simulink model "F16_dynamic_model_2019a"  (R2024b)
settings: Solver=ode3  StartTime=0.0  StopTime=1  FixedStep=1/1000  RelTol=1e-3
values from neighbouring files (symbols this model uses):
  f16data =     [f16aerodata.mat]
  f16engine =     [f16engine.mat]
undefined symbols (not defined in the file or in its folder): e0_0, e1_0, e2_0, e3_0, Earth, ft, m, s, WGS84
libraries: simulink_extras x11, simulink x7, aerosimlib x5, vrlib x3, sharedtransform x3, aerolibfltsims x3, slpidlib x3, aerolibconvert2 x2, aerolibutil x1, sharedutil x1, shared6dof x1, aerolibtransform2 x1
(part 1 of 3)
settings Model: SimulationMode=accelerator  PauseTimes=2  Creator=PC_2565  LastModifiedBy=MSI
settings SolverCC: AlgebraicLoopSolver=TrustRegion
settings DebuggingCC: UnconnectedInputMsg=warning  UnconnectedOutputMsg=warning  UnconnectedLineMsg=warning
settings ModelReferenceCC: EnableRefExpFcnMdlSchedulingChecks=on
settings SFSimCC: CustomCodeUndefinedFunction=UseInterfaceOnly
settings RTWCC: GPUComputeCapability=3.5

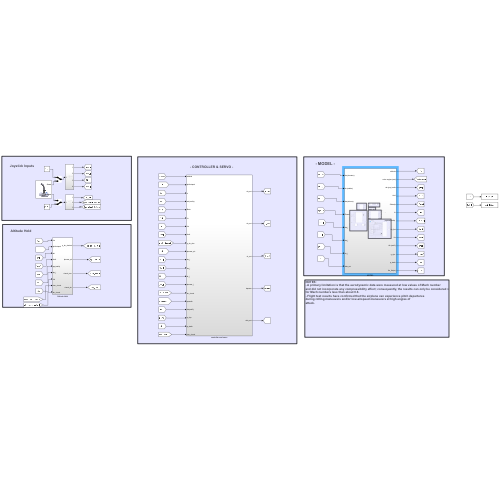
[thumbnail: Simulink's stored preview of the top-level diagram]
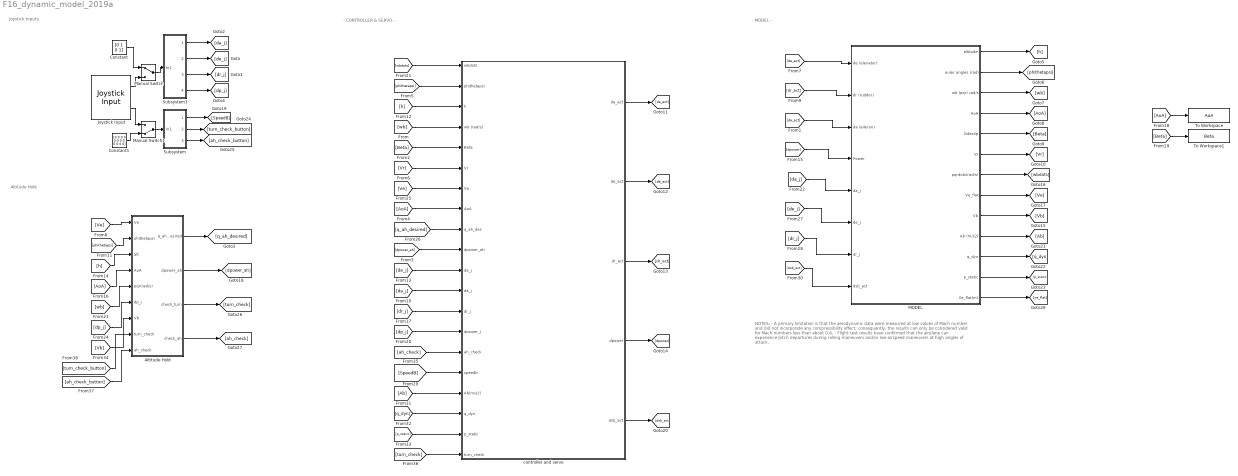
== system F16_dynamic_model_2019a ==
  note: NOTES:
      | - A primary limitation is that the aerodynamic data were measured at low values of Mach number
      | and did not incorporate any compressibility effect; consequently, the results can only be considered valid
      | for Mach numbers less than about 0.6.
      | - Flight test results have confirmed that the airplane can experience pitch departures
      | during rolling maneuvers and/or low-airspeed maneuvers at high angles of
      | attack.
  note: - CONTROLLER & SERVO -
  note: Altitude Hold
  note: Joystick Inputs
  note: - MODEL -
  Altitude Hold : Subsystem
  Constant : Constant  Value=[0 1 0 1]
  Constant1 : Constant  Value=[0 0 0 0 0 0 0 0 0 0 0 0]
  Joystick Input : vrlib/Joystick Input  joyid=1  adjustports=on  forcefeed=off
  MODEL : Subsystem
  Manual Switch : ManualSwitch
  Manual Switch1 : ManualSwitch  CurrentSetting=0
  Subsystem : Subsystem
  Subsystem3 : Subsystem
  To Workspace : ToWorkspace  VariableName=AoA  SampleTime=-1
  To Workspace1 : ToWorkspace  VariableName=Beta  SampleTime=-1
      settings: Save2DSignal=2-D array (concatenate along first dimension)
  "controller and servo " : Subsystem
  wires:
  Subsystem3/3(Out3) -> [dr_j]
  Subsystem3/4(Out4) -> [dp_j]
  MODEL/1(altitude) -> [h]
  MODEL/2(euler angles (rad)) -> [phithetapsi]
  MODEL/4(AoA) -> [AoA]
  MODEL/3(wb (pqr) rad/s) -> [wb]
  MODEL/5(Sideslip) -> [Beta]
  MODEL/6(Vr) -> [Vr]
  [phithetapsi] -> "controller and servo "/2(phithetapsi)
  "controller and servo "/1(da_act) -> [da_act]
  "controller and servo "/3(dr_act) -> [dr_act]
  [Vr] -> "controller and servo "/6(Vr)
  "controller and servo "/4(dpower) -> [dpower]
  [AoA] -> "controller and servo "/8(AoA)
  [h] -> "controller and servo "/3(h)
  [wb] -> "controller and servo "/4(wb (rad/s))
  MODEL/9(Vb) -> [Vb]
  [Ve] -> "controller and servo "/7(Ve)
  [Beta] -> "controller and servo "/5("Beta ")
  [AoA] -> To Workspace/1
  [Beta] -> To Workspace1/1
  [da_j] -> "controller and servo "/12(da_j)
  [de_j] -> "controller and servo "/11(de_j)
  [dr_j] -> "controller and servo "/13(dr_j)
  [dp_j] -> "controller and servo "/14(dpower_j)
  "controller and servo "/2(de_act) -> [de_act]
  [phithetapsi] -> Altitude Hold/2(phithetapsi)
  [h] -> Altitude Hold/3(alt)
  [AoA] -> Altitude Hold/4(AoA)
  [de_act] -> MODEL/1(de (elevator))
  [da_act] -> MODEL/3(da (aileron))
  [dr_act] -> MODEL/2(dr (rudder))
  [dpower] -> MODEL/4(Power)
  MODEL/7("pqrdots(rad/s) ") -> [wbdots]
  [wbdots] -> "controller and servo "/1(wbdots)
  [Ve] -> Altitude Hold/1(Ve)
  [wb] -> Altitude Hold/5(pqr(rad/s))
  [dp_j] -> Altitude Hold/6(dp_j)
  [ah_check] -> "controller and servo "/15("ah_check ")
  MODEL/8(Ve_flat) -> [Ve]
  Altitude Hold/1(q_ah_desired) -> [q_ah_desired]
  Altitude Hold/2(dpower_ah) -> [dpower_ah]
  [dpower_ah] -> "controller and servo "/10(dpower_ah)
  [q_ah_desired] -> "controller and servo "/9(q_ah_des)
  Joystick Input/1 -> Manual Switch/2
  Subsystem3/1(Out1) -> [da_j]
  Subsystem3/2(Out2) -> [de_j]
  [da_j] -> MODEL/5(da_j)
  [de_j] -> MODEL/6(de_j)
  [dr_j] -> MODEL/7(dr_j)
  [SpeedB] -> "controller and servo "/16(speedb)
  "controller and servo "/5(dsb_act) -> [dsb_act]
  [dsb_act] -> MODEL/8(dsb_act)
  MODEL/10(Ab (m/s2)) -> [Ab]
  [Ab] -> "controller and servo "/17(Ab(m/s2))
  MODEL/11("q_dyn ") -> [q_dyn]
  [q_dyn] -> "controller and servo "/18(q_dyn)
  MODEL/12(p_static) -> [p_static]
  [p_static] -> "controller and servo "/19(p_static)
  [Vb] -> Altitude Hold/7(Vb)
  Joystick Input/2 -> Manual Switch1/1
  Subsystem/1(Out1) -> [SpeedB]
  Subsystem/2(Out2) -> [turn_check_button]
  Subsystem/3(Out3) -> [ah_check_button]
  [turn_check] -> "controller and servo "/20("turn_check ")
  [turn_check_button] -> Altitude Hold/8("turn_check ")
  Altitude Hold/3("check_turn ") -> [turn_check]
  [ah_check_button] -> Altitude Hold/9(ah_check)
  Altitude Hold/4("check_ah ") -> [ah_check]
  Constant/1 -> Manual Switch/1
  Constant1/1 -> Manual Switch1/2
  MODEL/13(Xe_flat(m)) -> [xe_flat]
  Manual Switch1/1 -> Subsystem/1(In1)
  Manual Switch/1 -> Subsystem3/1(In1)

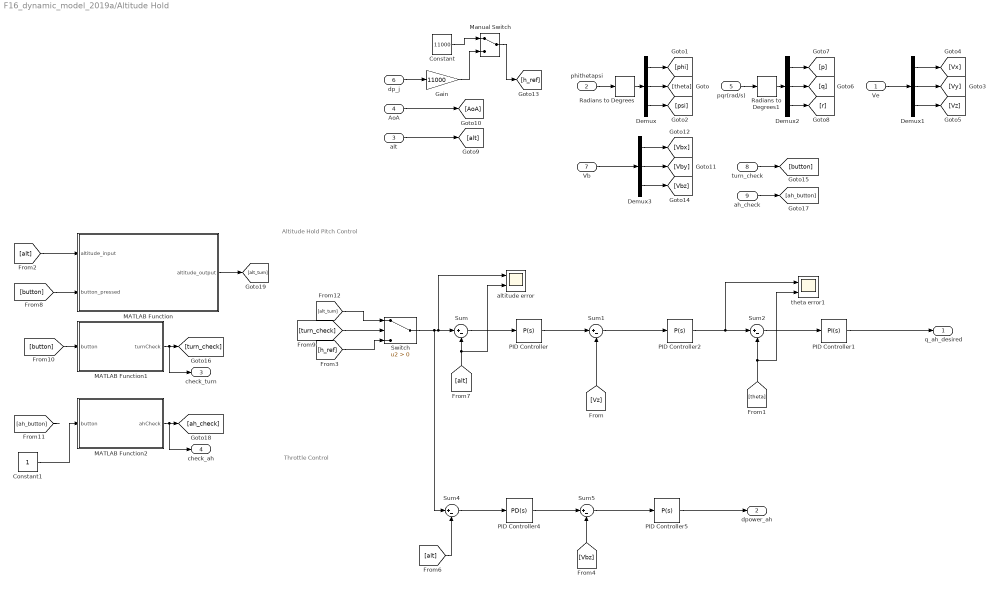
== system F16_dynamic_model_2019a/Altitude Hold ==
  note: Throttle Control
  note: Altitude Hold Pitch Control
  Ve : Inport
  phithetapsi : Inport  Port=2
  alt : Inport  Port=3
  AoA : Inport  Port=4
  pqr(rad/s) : Inport  Port=5
  dp_j : Inport  Port=6
  Vb : Inport  Port=7
  "turn_check " : Inport  Port=8
  ah_check : Inport  Port=9
  Constant : Constant  Value=11000
  Constant1 : Constant
  Demux{,1..3} (4 alike) : Demux  Outputs=3
  Gain : Gain  Gain=11000
  MATLAB Function : MATLAB Function  TreatAsAtomicUnit=on
  MATLAB Function1 : MATLAB Function  TreatAsAtomicUnit=on
  MATLAB Function2 : MATLAB Function  TreatAsAtomicUnit=on
  Manual Switch : ManualSwitch
  PID Controller : simulink/Continuous/PID Controller  Controller=P  Form=Parallel  TimeDomain=Continuous-time  SampleTime=-1  IntegratorMethod=Forward Euler  FilterMethod=Forward Euler  ControllerParametersSource=internal  P=2  I=0.00000001  D=10  UseFilter=on  N=100  TunerSelectOption=Transfer Function Based (PID Tuner App)  InitialConditionSource=internal  InitialConditionForIntegrator=0  InitialConditionForFilter=0  DifferentiatorICPrevScaledInput=0  ExternalReset=none  TrackingMode=off  Kt=1  LimitOutput=on  UpperSaturationLimit=254  LowerSaturationLimit=-254  LinearizeAsGain=on  AntiWindupMode=none  Kb=1  POutMin=[]  POutMax=[]  IOutMin=[]  IOutMax=[]  DOutMin=[]  DOutMax=[]  NOutMin=[]  NOutMax=[]  SumOutMin=[]  SumOutMax=[]  SaturationOutMin=[]  SaturationOutMax=[]  PParamMin=[]  PParamMax=[]  IParamMin=[]  IParamMax=[]  DParamMin=[]  DParamMax=[]  NParamMin=[]  NParamMax=[]  KbParamMin=[]  KbParamMax=[]  KtParamMin=[]  KtParamMax=[]  KbOutMin=[]  KbOutMax=[]  KtOutMin=[]  KtOutMax=[]  IntegratorOutMin=[]  IntegratorOutMax=[]  FilterOutMin=[]  FilterOutMax=[]  SumI1OutMin=[]  SumI1OutMax=[]  SumI2OutMin=[]  SumI2OutMax=[]  SumI3OutMin=[]  SumI3OutMax=[]  SumI4OutMin=[]  SumI4OutMax=[]  SumDOutMin=[]  SumDOutMax=[]  DifferentiatorOutMin=[]  DifferentiatorOutMax=[]  FilterDiffOutCoefMin=[]  FilterDiffOutCoefMax=[]  ReciprocalOutMin=[]  ReciprocalOutMax=[]  SumDenOutMin=[]  SumDenOutMax=[]  SumNumOutMin=[]  SumNumOutMax=[]  DivideOutMin=[]  DivideOutMax=[]  IntegratorContinuousStateAttributes=''  IntegratorStateMustResolveToSignalObject=off  IntegratorRTWStateStorageClass=Auto  FilterContinuousStateAttributes=''  FilterStateMustResolveToSignalObject=off  FilterRTWStateStorageClass=Auto  ParallelPVariant=InternalParameters  IdealPVariant=Disabled  IVariant=Disabled  DVariant=Disabled  IntegratorVariant=Disabled  SatVariant=Enabled  AWVariant=Disabled  PCopyVariant=Disabled  TRVariant=Disabled  FdbkBlocksVariant=Forward  IdealPFdbkVariant=Disabled  SatFdbkVariant=Disabled  DerivativeFilterVariant=Disabled  NVariant=Disabled  NCopyVariant=Disabled_SignalSpec  FilterICVariant=Disabled  IntegratorICVariant=Disabled  ExternalResetVariant=Disabled  TRSumVariant=Passthrough  SumFdbkVariant=Disabled  SumVariant=Passthrough_P
  PID Controller1 : simulink/Continuous/PID Controller  Controller=PI  Form=Parallel  TimeDomain=Continuous-time  SampleTime=-1  IntegratorMethod=Forward Euler  FilterMethod=Forward Euler  ControllerParametersSource=internal  P=0.1  I=0.01  D=10  UseFilter=on  N=100  TunerSelectOption=Transfer Function Based (PID Tuner App)  InitialConditionSource=internal  InitialConditionForIntegrator=0  InitialConditionForFilter=0  DifferentiatorICPrevScaledInput=0  ExternalReset=none  TrackingMode=off  Kt=1  LimitOutput=on  UpperSaturationLimit=inf  LowerSaturationLimit=-inf  LinearizeAsGain=on  AntiWindupMode=clamping  Kb=1  POutMin=[]  POutMax=[]  IOutMin=[]  IOutMax=[]  DOutMin=[]  DOutMax=[]  NOutMin=[]  NOutMax=[]  SumOutMin=[]  SumOutMax=[]  SaturationOutMin=[]  SaturationOutMax=[]  PParamMin=[]  PParamMax=[]  IParamMin=[]  IParamMax=[]  DParamMin=[]  DParamMax=[]  NParamMin=[]  NParamMax=[]  KbParamMin=[]  KbParamMax=[]  KtParamMin=[]  KtParamMax=[]  KbOutMin=[]  KbOutMax=[]  KtOutMin=[]  KtOutMax=[]  IntegratorOutMin=[]  IntegratorOutMax=[]  FilterOutMin=[]  FilterOutMax=[]  SumI1OutMin=[]  SumI1OutMax=[]  SumI2OutMin=[]  SumI2OutMax=[]  SumI3OutMin=[]  SumI3OutMax=[]  SumI4OutMin=[]  SumI4OutMax=[]  SumDOutMin=[]  SumDOutMax=[]  DifferentiatorOutMin=[]  DifferentiatorOutMax=[]  FilterDiffOutCoefMin=[]  FilterDiffOutCoefMax=[]  ReciprocalOutMin=[]  ReciprocalOutMax=[]  SumDenOutMin=[]  SumDenOutMax=[]  SumNumOutMin=[]  SumNumOutMax=[]  DivideOutMin=[]  DivideOutMax=[]  IntegratorContinuousStateAttributes=''  IntegratorStateMustResolveToSignalObject=off  IntegratorRTWStateStorageClass=Auto  FilterContinuousStateAttributes=''  FilterStateMustResolveToSignalObject=off  FilterRTWStateStorageClass=Auto  ParallelPVariant=InternalParameters  IdealPVariant=Disabled  IVariant=InternalParameters  DVariant=Disabled  IntegratorVariant=Continuous  SatVariant=Enabled  AWVariant=ContClampingParallel  PCopyVariant=Disabled  TRVariant=Disabled  FdbkBlocksVariant=Forward  IdealPFdbkVariant=Disabled  SatFdbkVariant=Disabled  DerivativeFilterVariant=Disabled  NVariant=Disabled  NCopyVariant=Disabled_SignalSpec  FilterICVariant=Disabled  IntegratorICVariant=InternalICs  ExternalResetVariant=Disabled  TRSumVariant=Passthrough  SumFdbkVariant=Disabled  SumVariant=Sum_PI
  PID Controller2 : simulink/Continuous/PID Controller  Controller=P  Form=Parallel  TimeDomain=Continuous-time  SampleTime=-1  IntegratorMethod=Forward Euler  FilterMethod=Forward Euler  ControllerParametersSource=internal  P=2  I=0.001  D=0.1  UseFilter=on  N=100  TunerSelectOption=Transfer Function Based (PID Tuner App)  InitialConditionSource=internal  InitialConditionForIntegrator=0  InitialConditionForFilter=0  DifferentiatorICPrevScaledInput=0  ExternalReset=none  TrackingMode=off  Kt=1  LimitOutput=on  UpperSaturationLimit=45  LowerSaturationLimit=-45  LinearizeAsGain=on  AntiWindupMode=none  Kb=1  POutMin=[]  POutMax=[]  IOutMin=[]  IOutMax=[]  DOutMin=[]  DOutMax=[]  NOutMin=[]  NOutMax=[]  SumOutMin=[]  SumOutMax=[]  SaturationOutMin=[]  SaturationOutMax=[]  PParamMin=[]  PParamMax=[]  IParamMin=[]  IParamMax=[]  DParamMin=[]  DParamMax=[]  NParamMin=[]  NParamMax=[]  KbParamMin=[]  KbParamMax=[]  KtParamMin=[]  KtParamMax=[]  KbOutMin=[]  KbOutMax=[]  KtOutMin=[]  KtOutMax=[]  IntegratorOutMin=[]  IntegratorOutMax=[]  FilterOutMin=[]  FilterOutMax=[]  SumI1OutMin=[]  SumI1OutMax=[]  SumI2OutMin=[]  SumI2OutMax=[]  SumI3OutMin=[]  SumI3OutMax=[]  SumI4OutMin=[]  SumI4OutMax=[]  SumDOutMin=[]  SumDOutMax=[]  DifferentiatorOutMin=[]  DifferentiatorOutMax=[]  FilterDiffOutCoefMin=[]  FilterDiffOutCoefMax=[]  ReciprocalOutMin=[]  ReciprocalOutMax=[]  SumDenOutMin=[]  SumDenOutMax=[]  SumNumOutMin=[]  SumNumOutMax=[]  DivideOutMin=[]  DivideOutMax=[]  IntegratorContinuousStateAttributes=''  IntegratorStateMustResolveToSignalObject=off  IntegratorRTWStateStorageClass=Auto  FilterContinuousStateAttributes=''  FilterStateMustResolveToSignalObject=off  FilterRTWStateStorageClass=Auto  ParallelPVariant=InternalParameters  IdealPVariant=Disabled  IVariant=Disabled  DVariant=Disabled  IntegratorVariant=Disabled  SatVariant=Enabled  AWVariant=Disabled  PCopyVariant=Disabled  TRVariant=Disabled  FdbkBlocksVariant=Forward  IdealPFdbkVariant=Disabled  SatFdbkVariant=Disabled  DerivativeFilterVariant=Disabled  NVariant=Disabled  NCopyVariant=Disabled_SignalSpec  FilterICVariant=Disabled  IntegratorICVariant=Disabled  ExternalResetVariant=Disabled  TRSumVariant=Passthrough  SumFdbkVariant=Disabled  SumVariant=Passthrough_P
  PID Controller4 : simulink/Continuous/PID Controller  Controller=PD  Form=Parallel  TimeDomain=Continuous-time  SampleTime=-1  IntegratorMethod=Forward Euler  FilterMethod=Forward Euler  ControllerParametersSource=internal  P=5  I=0.00000001  D=10  UseFilter=on  N=100  TunerSelectOption=Transfer Function Based (PID Tuner App)  InitialConditionSource=internal  InitialConditionForIntegrator=0  InitialConditionForFilter=0  DifferentiatorICPrevScaledInput=0  ExternalReset=none  TrackingMode=off  Kt=1  LimitOutput=on  UpperSaturationLimit=254  LowerSaturationLimit=-254  LinearizeAsGain=on  AntiWindupMode=none  Kb=1  POutMin=[]  POutMax=[]  IOutMin=[]  IOutMax=[]  DOutMin=[]  DOutMax=[]  NOutMin=[]  NOutMax=[]  SumOutMin=[]  SumOutMax=[]  SaturationOutMin=[]  SaturationOutMax=[]  PParamMin=[]  PParamMax=[]  IParamMin=[]  IParamMax=[]  DParamMin=[]  DParamMax=[]  NParamMin=[]  NParamMax=[]  KbParamMin=[]  KbParamMax=[]  KtParamMin=[]  KtParamMax=[]  KbOutMin=[]  KbOutMax=[]  KtOutMin=[]  KtOutMax=[]  IntegratorOutMin=[]  IntegratorOutMax=[]  FilterOutMin=[]  FilterOutMax=[]  SumI1OutMin=[]  SumI1OutMax=[]  SumI2OutMin=[]  SumI2OutMax=[]  SumI3OutMin=[]  SumI3OutMax=[]  SumI4OutMin=[]  SumI4OutMax=[]  SumDOutMin=[]  SumDOutMax=[]  DifferentiatorOutMin=[]  DifferentiatorOutMax=[]  FilterDiffOutCoefMin=[]  FilterDiffOutCoefMax=[]  ReciprocalOutMin=[]  ReciprocalOutMax=[]  SumDenOutMin=[]  SumDenOutMax=[]  SumNumOutMin=[]  SumNumOutMax=[]  DivideOutMin=[]  DivideOutMax=[]  IntegratorContinuousStateAttributes=''  IntegratorStateMustResolveToSignalObject=off  IntegratorRTWStateStorageClass=Auto  FilterContinuousStateAttributes=''  FilterStateMustResolveToSignalObject=off  FilterRTWStateStorageClass=Auto  ParallelPVariant=InternalParameters  IdealPVariant=Disabled  IVariant=Disabled  DVariant=InternalParameters  IntegratorVariant=Disabled  SatVariant=Enabled  AWVariant=Disabled  PCopyVariant=Disabled  TRVariant=Disabled  FdbkBlocksVariant=Forward  IdealPFdbkVariant=Disabled  SatFdbkVariant=Disabled  DerivativeFilterVariant=ContFilter  NVariant=InternalParameters  NCopyVariant=Disabled  FilterICVariant=InternalICsFilter  IntegratorICVariant=Disabled  ExternalResetVariant=Disabled  TRSumVariant=Passthrough  SumFdbkVariant=Disabled  SumVariant=Sum_PD
  PID Controller5 : simulink/Continuous/PID Controller  Controller=P  Form=Parallel  TimeDomain=Continuous-time  SampleTime=-1  IntegratorMethod=Forward Euler  FilterMethod=Forward Euler  ControllerParametersSource=internal  P=10  I=0.00001  D=0.01  UseFilter=on  N=100  TunerSelectOption=Transfer Function Based (PID Tuner App)  InitialConditionSource=internal  InitialConditionForIntegrator=0  InitialConditionForFilter=0  DifferentiatorICPrevScaledInput=0  ExternalReset=none  TrackingMode=off  Kt=1  LimitOutput=on  UpperSaturationLimit=1  LowerSaturationLimit=0  LinearizeAsGain=on  AntiWindupMode=none  Kb=1  POutMin=[]  POutMax=[]  IOutMin=[]  IOutMax=[]  DOutMin=[]  DOutMax=[]  NOutMin=[]  NOutMax=[]  SumOutMin=[]  SumOutMax=[]  SaturationOutMin=[]  SaturationOutMax=[]  PParamMin=[]  PParamMax=[]  IParamMin=[]  IParamMax=[]  DParamMin=[]  DParamMax=[]  NParamMin=[]  NParamMax=[]  KbParamMin=[]  KbParamMax=[]  KtParamMin=[]  KtParamMax=[]  KbOutMin=[]  KbOutMax=[]  KtOutMin=[]  KtOutMax=[]  IntegratorOutMin=[]  IntegratorOutMax=[]  FilterOutMin=[]  FilterOutMax=[]  SumI1OutMin=[]  SumI1OutMax=[]  SumI2OutMin=[]  SumI2OutMax=[]  SumI3OutMin=[]  SumI3OutMax=[]  SumI4OutMin=[]  SumI4OutMax=[]  SumDOutMin=[]  SumDOutMax=[]  DifferentiatorOutMin=[]  DifferentiatorOutMax=[]  FilterDiffOutCoefMin=[]  FilterDiffOutCoefMax=[]  ReciprocalOutMin=[]  ReciprocalOutMax=[]  SumDenOutMin=[]  SumDenOutMax=[]  SumNumOutMin=[]  SumNumOutMax=[]  DivideOutMin=[]  DivideOutMax=[]  IntegratorContinuousStateAttributes=''  IntegratorStateMustResolveToSignalObject=off  IntegratorRTWStateStorageClass=Auto  FilterContinuousStateAttributes=''  FilterStateMustResolveToSignalObject=off  FilterRTWStateStorageClass=Auto  ParallelPVariant=InternalParameters  IdealPVariant=Disabled  IVariant=Disabled  DVariant=Disabled  IntegratorVariant=Disabled  SatVariant=Enabled  AWVariant=Disabled  PCopyVariant=Disabled  TRVariant=Disabled  FdbkBlocksVariant=Forward  IdealPFdbkVariant=Disabled  SatFdbkVariant=Disabled  DerivativeFilterVariant=Disabled  NVariant=Disabled  NCopyVariant=Disabled_SignalSpec  FilterICVariant=Disabled  IntegratorICVariant=Disabled  ExternalResetVariant=Disabled  TRSumVariant=Passthrough  SumFdbkVariant=Disabled  SumVariant=Passthrough_P
  Radians to Degrees : simulink_extras/Transformations/Radians to Degrees
  Radians to Degrees1 : simulink_extras/Transformations/Radians to Degrees
  Sum{,1..2,4..5} (5 alike) : Sum  Inputs=|+-
  Switch : Switch  Criteria=u2 > Threshold  SaturateOnIntegerOverflow=off  InputSameDT=off
  altitude error : Scope  NumInputPorts=2
  theta error1 : Scope  NumInputPorts=2
  q_ah_desired : Outport
  dpower_ah : Outport  Port=2
  "check_turn " : Outport  Port=3
  "check_ah " : Outport  Port=4
  wires:
  Sum/1 -> PID Controller/1
  Demux/2 -> [theta]
  Demux/3 -> [psi]
  Demux/1 -> [phi]
  phithetapsi/1 -> Radians to Degrees/1
  Radians to Degrees/1 -> Demux/1
  alt/1 -> [alt]
  Demux1/1 -> [Vx]
  Demux1/2 -> [Vy]
  Demux1/3 -> [Vz]
  Ve/1 -> Demux1/1
  Demux2/2 -> [q]
  Demux2/1 -> [p]
  Radians to Degrees1/1 -> Demux2/1
  Demux2/3 -> [r]
  pqr(rad/s)/1 -> Radians to Degrees1/1
  PID Controller5/1 -> dpower_ah/1
  PID Controller4/1 -> Sum5/1
  Sum5/1 -> PID Controller5/1
  [Vbz] -> Sum5/2
  Sum4/1 -> PID Controller4/1
  [alt] -> Sum4/2
  dp_j/1 -> Gain/1
  Gain/1 -> Manual Switch/2
  AoA/1 -> [AoA]
  [alt] -> altitude error/2, Sum/2
  PID Controller/1 -> Sum1/1
  Sum1/1 -> PID Controller2/1
  Constant/1 -> Manual Switch/1
  Manual Switch/1 -> [h_ref]
  Demux3/1 -> [Vbx]
  Demux3/2 -> [Vby]
  Demux3/3 -> [Vbz]
  Vb/1 -> Demux3/1
  [Vz] -> Sum1/2
  PID Controller2/1 -> theta error1/1, Sum2/1
  [theta] -> theta error1/2, Sum2/2
  Sum2/1 -> PID Controller1/1
  PID Controller1/1 -> q_ah_desired/1
  [alt] -> MATLAB Function/1(altitude_input)
  "turn_check "/1 -> [button]
  [button] -> MATLAB Function/2(button_pressed)
  MATLAB Function/1(altitude_output) -> [alt_turn]
  MATLAB Function1/1(turnCheck) -> "check_turn "/1, [turn_check]
  [button] -> MATLAB Function1/1(button)
  [turn_check] -> Switch/2
  [h_ref] -> Switch/3
  Switch/1 -> altitude error/1, Sum/1, Sum4/1
  ah_check/1 -> [ah_button]
  [ah_button] -> ?
  MATLAB Function2/1(ahCheck) -> "check_ah "/1, [ah_check]
  [alt_turn] -> Switch/1
  Constant1/1 -> MATLAB Function2/1(button)

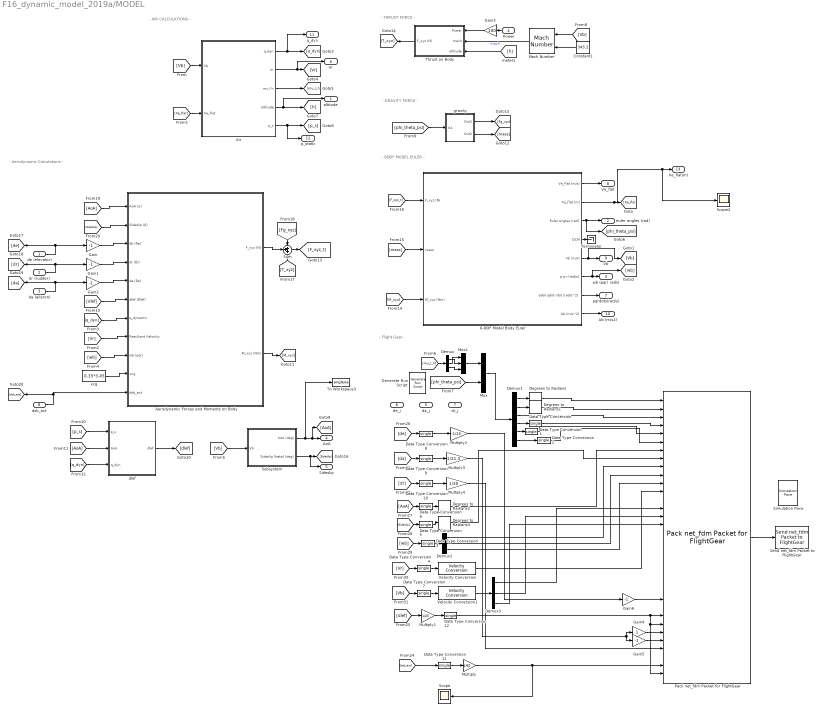
== system F16_dynamic_model_2019a/MODEL ==
  note: - Aerodynamic Calculations -
  note: - AIR CALCULATIONS -
  note: - Flight Gear -
  note: - 6DOF MODEL EULER -
  note: - GRAVITY FORCE -
  note: - THRUST FORCE -
  de (elevator) : Inport
  dr (rudder) : Inport  Port=2
  da (aileron) : Inport  Port=3
  Power : Inport  Port=4
  da_j : Inport  Port=5
  de_j : Inport  Port=6
  dr_j : Inport  Port=7
  dsb_act : Inport  Port=8
  6-DOF Model Body Euler : Subsystem
  Aerodynamic Forces and Moments on Body : Subsystem
  "Air " : Subsystem
  Constant1 : Constant  Value=343.2
  Data Type Conversion{,1..12} (13 alike) : DataTypeConversion  OutDataTypeStr=single  SaturateOnIntegerOverflow=off  RndMeth=Floor
  Degrees to Radians{,1..3} (4 alike) : simulink_extras/Transformations/Degrees to Radians
  Demux : Demux  Outputs=3
  Demux1 : Demux  Outputs=6
  Demux2 : Demux  Outputs=3
  Demux3 : Demux  Outputs=3
  Gain{,1..2,5..6} (5 alike) : Gain  Gain=-1
  Gain3 : Gain  Gain=100
  Gain4 : Gain
  Generate Run Script : aerolibfltsims/Generate Run Script  Architecture=Default  dataFlow=Send  GeometryModelName=c172p  AirportId=KSFO  RunwayId=10L  InitialAltitude=7224  InitialHeading=113  OffsetDistance=4.72  OffsetAzimuth=0  InstallScenery=off  DisableShaders=off  OriginAddress=127.0.0.1  DestinationPort=5502  OriginPort=5505  LocalAddress=127.0.0.1  OutputFileName=runfg.bat  FlightGearBaseDirectory=C:\Program Files\FlightGear 2020.3
  Mach Number : aerolibasang/Mach Number
  Multiply : Gain  Gain=1/60
  Multiply1 : Gain  Gain=1/25
  Multiply2 : Gain  Gain=-1/25
  Multiply3 : Gain  Gain=1/21.5
  Multiply4 : Gain  Gain=1/30
  Mux : Mux  Inputs=2
  Mux1 : Mux  Inputs=3
  Pack net_fdm Packet for FlightGear : aerolibfltsims/Pack net_fdm Packet for FlightGear  FlightGearVersion=v2018.3  ShowPositionAttitudeInputs=on  ShowVelocityAccelerationInputs=on  ShowControlSurfacePositionInputs=on  ShowEngineFuelInputs=off  ShowLandingGearInputs=off  ShowEnvironmentInputs=off  SampleTime=1/50  packetVersion=24
  Scope : Scope
  Scope2 : Scope
  Send net_fdm Packet to FlightGear : aerolibfltsims/Send net_fdm Packet to FlightGear  DestinationIpAddress=127.0.0.1  DestinationPort=5502  LocalIpPort=-1  varLen=off  SampleTime=1/50
  Simulation Pace : aerolibanimutils/Simulation Pace  SimulationPace=1  SleepMode=MATLAB Thread  OutputPaceError=off  SampleTime=1/50
      settings: AttributesFormatString=%<SimulationPace> sec/sec
  Subsystem : Subsystem
  Sum : Sum  Inputs=+++
  Terminator : Terminator
  "Thrust on Body " : Subsystem
  To Workspace3 : ToWorkspace  VariableName=angleoa  SampleTime=-1
  Velocity Conversion : aerolibconvert2/Velocity Conversion  IU=m/s  OU=kts
  Velocity Conversion1 : aerolibconvert2/Velocity Conversion  IU=m/s  OU=ft/s
  dlef : Subsystem
  gravity : Subsystem
  xcg : Constant  Value=0.35*3.45
  altitude : Outport
  euler angles (rad) : Outport  Port=2
  wb (pqr) rad/s : Outport  Port=3
  AoA : Outport  Port=4
  Sideslip : Outport  Port=5
  Vr : Outport  Port=6
  "pqrdots(rad/s) " : Outport  Port=7
  Ve_flat : Outport  Port=8
  Vb : Outport  Port=9
  Ab (m/s2) : Outport  Port=10
  "q_dyn " : Outport  Port=11
  p_static : Outport  Port=12
  Xe_flat(m) : Outport  Port=13
  wires:
  [mu_I_h] -> Demux/1
  [wb] -> Aerodynamic Forces and Moments on Body/9(wb (pqr))
  6-DOF Model Body Euler/6(p q r (rad/s)) -> [wb], wb (pqr) rad/s/1
  [Vr] -> Aerodynamic Forces and Moments on Body/8(Resultant Velocity)
  Aerodynamic Forces and Moments on Body/1(F_xyz (N)) -> Sum/2
  Subsystem/2(Sideslip (beta) (deg)) -> Sideslip/1, [Sideslip]
  Mach Number/1 -> "Thrust on Body "/2(mach)  "mach"
  "Air "/1("q_dyn ") -> "q_dyn "/1, [q_dyn]
  "Air "/4("altitude ") -> [h], altitude/1
  [phi_theta_psi] -> Mux/2
  Constant1/1 -> Mach Number/2
  "Air "/2(Vr) -> Vr/1, [Vr]
  [Xe_flat] -> "Air "/2(Xe_flat)
  6-DOF Model Body Euler/4(DCM) -> Terminator/1
  [q_dyn] -> Aerodynamic Forces and Moments on Body/7(q_dynamic)
  6-DOF Model Body Euler/8(Ab (m/s^2)) -> Ab (m/s2)/1
  6-DOF Model Body Euler/1(Ve_flat (m/s)) -> Ve_flat/1
  6-DOF Model Body Euler/3(Euler Angles (rad)) -> [phi_theta_psi], euler angles (rad)/1
  6-DOF Model Body Euler/2(Xe_flat (m)) -> Scope2/1, Xe_flat(m)/1, [Xe_flat]
  [Vb] -> Mach Number/1
  "Air "/3(mu I h) -> [mu_I_h]
  xcg/1 -> Aerodynamic Forces and Moments on Body/10("xcg ")
  [Vb] -> Subsystem/1(Vb)
  [Vb] -> "Air "/1(Vb)
  6-DOF Model Body Euler/7(pdot qdot rdot (rad/s^2)) -> "pqrdots(rad/s) "/1
  Demux/1 -> Mux1/2
  Demux/2 -> Mux1/1
  Demux/3 -> Mux1/3
  Mux1/1 -> Mux/1
  Gain3/1 -> "Thrust on Body "/1(Power)
  Power/1 -> Gain3/1
  [phi_theta_psi] -> gravity/1(In1)
  Subsystem/1(AoA (deg)) -> To Workspace3/1, [AoA], AoA/1
  "Air "/5(p_s) -> p_static/1, [p_s]
  [p_s] -> dlef/1("p_s ")
  [AoA] -> dlef/2(AoA)
  [q_dyn] -> dlef/3("q_dyn ")
  dlef/1(dlef) -> [dlef]
  [dlef] -> Aerodynamic Forces and Moments on Body/6(dlef (δlef))
  Aerodynamic Forces and Moments on Body/2(M_xyz (Nm)) -> [M_xyz]
  [M_xyz] -> 6-DOF Model Body Euler/3(M_xyz (Nm))
  gravity/2(Out2) -> [mass]
  [mass] -> 6-DOF Model Body Euler/2(mass)
  Sum/1 -> [F_xyz_t]
  [F_xyz_t] -> 6-DOF Model Body Euler/1(F_xyz (N))
  [T_xyz] -> Sum/3
  gravity/1(Out1) -> [Fg_xyz]
  [Fg_xyz] -> Sum/1
  6-DOF Model Body Euler/5(Vb (m/s)) -> Vb/1, [Vb]
  [Sideslip] -> Aerodynamic Forces and Moments on Body/2(Sideslip (β))
  [AoA] -> Aerodynamic Forces and Moments on Body/1(AoA (α))
  [h] -> "Thrust on Body "/3(altitude)
  de (elevator)/1 -> [de], Gain/1
  Gain/1 -> Aerodynamic Forces and Moments on Body/3(dh (δe))
  dr (rudder)/1 -> [dr], Gain1/1
  da (aileron)/1 -> Gain2/1, [da]
  Gain1/1 -> Aerodynamic Forces and Moments on Body/4(dr (δr))
  Gain2/1 -> Aerodynamic Forces and Moments on Body/5(da (δa))
  "Thrust on Body "/1(F_xyz (N)) -> [T_xyz]
  Pack net_fdm Packet for FlightGear/1 -> Send net_fdm Packet to FlightGear/1
  Demux1/1 -> Degrees to Radians/1
  Demux1/2 -> Degrees to Radians1/1
  Demux1/3 -> Pack net_fdm Packet for FlightGear/3
  Demux1/4 -> Data Type Conversion/1
  Demux1/5 -> Data Type Conversion1/1
  Demux1/6 -> Data Type Conversion2/1
  Mux/1 -> Demux1/1
  Degrees to Radians/1 -> Pack net_fdm Packet for FlightGear/1
  Degrees to Radians1/1 -> Pack net_fdm Packet for FlightGear/2
  [AoA] -> Data Type Conversion6/1
  Degrees to Radians2/1 -> Pack net_fdm Packet for FlightGear/7
  [Sideslip] -> Data Type Conversion5/1
  Degrees to Radians3/1 -> Pack net_fdm Packet for FlightGear/8
  [wb] -> Data Type Conversion3/1
  Demux2/1 -> Pack net_fdm Packet for FlightGear/9
  Demux2/2 -> Pack net_fdm Packet for FlightGear/10
  Demux2/3 -> Pack net_fdm Packet for FlightGear/11
  [Vr] -> Data Type Conversion4/1
  Velocity Conversion/1 -> Pack net_fdm Packet for FlightGear/12
  [Vb] -> Data Type Conversion7/1
  Velocity Conversion1/1 -> Demux3/1
  Demux3/1 -> Pack net_fdm Packet for FlightGear/14
  Demux3/2 -> Pack net_fdm Packet for FlightGear/15
  Demux3/3 -> Pack net_fdm Packet for FlightGear/16
  Data Type Conversion8/1 -> Multiply2/1
  Data Type Conversion10/1 -> Multiply4/1
  Data Type Conversion/1 -> Pack net_fdm Packet for FlightGear/4
  Data Type Conversion1/1 -> Pack net_fdm Packet for FlightGear/5
  Data Type Conversion2/1 -> Pack net_fdm Packet for FlightGear/6
  Data Type Conversion3/1 -> Demux2/1
  Data Type Conversion4/1 -> Velocity Conversion/1
  Data Type Conversion5/1 -> Degrees to Radians3/1
  Data Type Conversion6/1 -> Degrees to Radians2/1
  Data Type Conversion7/1 -> Velocity Conversion1/1
  [dsb_act] -> Data Type Conversion11/1
  Data Type Conversion11/1 -> Multiply/1
  dsb_act/1 -> Aerodynamic Forces and Moments on Body/11("dsb_act "), [dsb_act]
  Multiply/1 -> Scope/1, Pack net_fdm Packet for FlightGear/33
  Data Type Conversion9/1 -> Multiply3/1
  Gain4/1 -> Pack net_fdm Packet for FlightGear/29
  Gain5/1 -> Pack net_fdm Packet for FlightGear/30
  Gain6/1 -> Pack net_fdm Packet for FlightGear/25
  [dlef] -> Multiply1/1
  Data Type Conversion12/1 -> Pack net_fdm Packet for FlightGear/34, Pack net_fdm Packet for FlightGear/28, Pack net_fdm Packet for FlightGear/27
  Multiply1/1 -> Data Type Conversion12/1
  [de] -> Data Type Conversion8/1
  Multiply2/1 -> Gain6/1
  [dr] -> Data Type Conversion10/1
  [da] -> Data Type Conversion9/1
  Multiply3/1 -> Gain5/1, Gain4/1
  Multiply4/1 -> Pack net_fdm Packet for FlightGear/31

== system F16_dynamic_model_2019a/Subsystem ==
  In1 : Inport
  Data Type Conversion : DataTypeConversion  OutDataTypeStr=double  SaturateOnIntegerOverflow=off  RndMeth=Floor
  Demux : Demux  Outputs=3
  Selector : Selector  InputPortWidth=12  IndexOptions=Index vector (dialog)  Indices=[1 2 3]  OutputSizes=1
  Out1 : Outport
  Out2 : Outport  Port=2
  Out3 : Outport  Port=3
  wires:
  Demux/1 -> Data Type Conversion/1
  Selector/1 -> Demux/1
  In1/1 -> Selector/1
  Data Type Conversion/1 -> Out1/1
  Demux/2 -> Out2/1
  Demux/3 -> Out3/1

== system F16_dynamic_model_2019a/Subsystem3 ==
  In1 : Inport
  Demux : Demux
  Subsystem2 : Subsystem
  Out1 : Outport
  Out2 : Outport  Port=2
  Out3 : Outport  Port=3
  Out4 : Outport  Port=4
  wires:
  Demux/4 -> Subsystem2/1(In1)
  In1/1 -> Demux/1
  Demux/2 -> Out2/1
  Demux/3 -> Out3/1
  Subsystem2/1(Out1) -> Out4/1
  Demux/1 -> Out1/1
